simulink model "TBRe18_ECU_V6"  (R2015b)
settings: Solver=FixedStepDiscrete  SolverMode=SingleTasking  StartTime=0.0  StopTime=inf  FixedStep=0.0001  RelTol=1e-3
PostLoadFcn:
  | model_init();
libraries: simulink x20, simulink_extras x1
(part 1 of 4)
settings Model: Creator=agf25  LastModifiedBy=William
settings OptimizationCC: DefaultParameterBehavior=Inlined  EfficientFloat2IntCast=on
settings RTWCC: SystemTargetFile=nsi_mpc.tlc  MakeCommand=nsi_make  TemplateMakefile=nsi_mpc.tmf  Description=RTW Coder for MUXLAB4
settings STFCustomTargetCC: ConcurrentExecutionCompliant=off  GeneratePreprocessorConditionals=Use local settings  MATLABClassNameForMDSCustomization=Simulink.SoftwareTarget.TargetSpecificTriggerConfigurationBase  CPPClassGenCompliant=off  SystemTargetFile=nsi_mpc.tlc

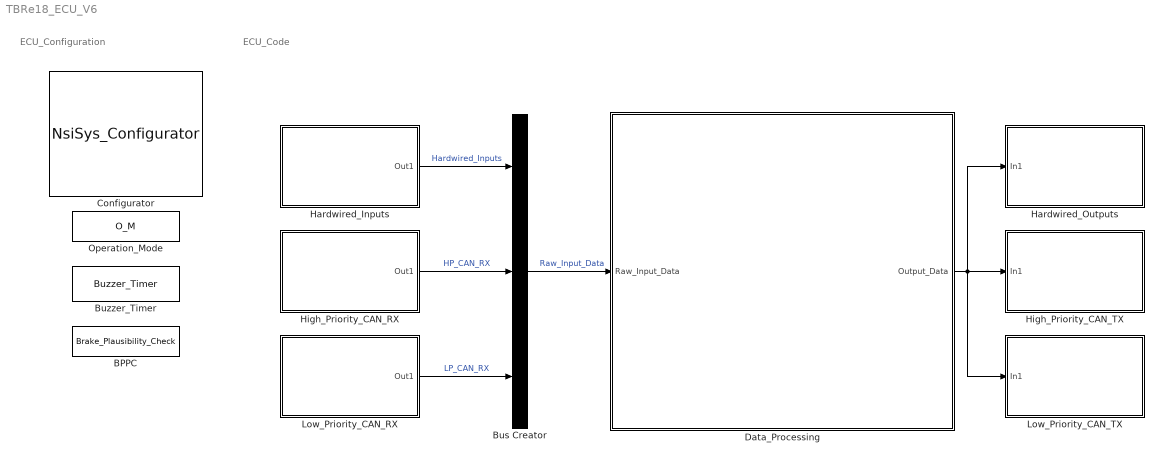
== system TBRe18_ECU_V6 ==
  note: ECU_Code
  note: ECU_Configuration
  BPPC : DataStoreMemory  DataStoreName=Brake_Plausibility_Check  ReadBeforeWriteMsg=warning  WriteAfterWriteMsg=warning  WriteAfterReadMsg=warning  OutDataTypeStr=boolean
  Bus Creator : BusCreator  Inputs=3
  Buzzer_Timer : DataStoreMemory  DataStoreName=Buzzer_Timer  ReadBeforeWriteMsg=warning  WriteAfterWriteMsg=warning  WriteAfterReadMsg=warning
  Configurator : S-Function  FunctionName=NsiSys_Configurator  Parameters=main,io,nbof_can,can,ccp,flash,nbof_lin,lin,tasks  SFunctionDeploymentMode=off  EnableBusSupport=off  mask(Configurator block){main=Config description;01/01/2011;0, io=2.5;0;1;1;0;0;1;1;1, nbof_can=5, can=1;HIGH_SPEED;500Kbps;120 Ohm;C:\Users\William\Documents\ECU\DBC\TBRe18_DBC_V1.dbc;0;1;1;HIGH_SPEED;500Kbps;120 Ohm;C:\Users\William\Documents\ECU\DBC\TBRe18_DBC_V1.dbc;0;1;0;HIGH_SPEED;500Kbps;120 Ohm;C:\Users\l\Desktop\FYP\ECU\DBC\TBRe_DBC_V2.dbc;0;0;0;HIGH_SPEED;500Kbps;120 Ohm;D:\TOOLS\MUXLINK\R2011b\MUXlink\misc\j1939_adapt.dbc;0;1;0;HIGH_SPEED;1000Kbps;No;D:\TOOLS\MUXLINK\R2011b\MUXlink\misc\BASE_CAN_MUXLAB4.dbc;0;0, ccp=0;0x100;0x200;0;0;0x0;0x0;0;0x13, flash=Vehicle_STATE;No;Unsigned Byte;0;1;Operational_STATE;No;Unsigned Byte;0;1;Buzzer_time;No;Unsigned Byte;254;1;Buzzer_on;No;Boolean;1;1;reset_MEM;No;Boolean;0;1;TC_Slip_target;No;Unsigned Byte;5;1;TC_P_Gain;No;Unsigned Byte;1;1;TC_I_Gain;No;Unsigned Byte;1;1;TC_Offset;No;Signed Byte;0;1;DM_Mode;No;Unsigned Byte;0;1;DM_I_Gain;No;Unsigned Byte;1;1;IMD_MEM;No;Boolean;0;1;status_vehcle_LV;No;Boolean;0;1;status_vehcle_HV;No;Boolean;0;1;status_BMS;No;Boolean;0;1;status_IMD;No;Boolean;0;1;status_APPC;No;Boolean;0;1;status_APPS_BPPC;No;Boolean;0;1;status_RTD;No;Boolean;0;1;status_TC;No;Boolean;0;1;status_power_lim;No;Boolean;0;1;status_torque_derate;No;Boolean;0;1;status_tyre_radius;No;Unsigned Byte;22;1;power_limit;No;Unsigned Byte;30;1;torque_limit;No;Unsigned Byte;80;1, nbof_lin=2, lin=0;D:\TOOLS\MUXLINK\R2011b\MUXlink\misc\lindb.ldf;1;0.0;0.0;0.000;0.000;0.000000;0,0;0;D:\TOOLS\MUXLINK\R2011b\MUXlink\misc\lindb.ldf;1;0.0;0.0;0.000;0.000;0.000000;0,0, tasks=Data_Processing;[0.100];Hardwired_Inputs;[0.1];Hardwired_Outputs;[0.1];High_Priority_CAN_RX;[0.1];High_Priority_CAN_TX;[0.1];Low_Priority_CAN_RX;[0.1];Low_Priority_CAN_TX;[0.1]}
      mask prompts: nbof_can "nbof can"
      mask help: This block permits to set general parameters to use a MUXlink model
      mask init:
      | NsiSys_Configurator_InitializationFcn();
      settings: OpenFcn=NsiSys_Configurator_OpenFcn();
      mask Help:
      | eval('block=get_param(gcb, ''RTWdata'');')
      | web([docroot '\toolbox\MUXlink\html\blocks/' block.MUXlink_BlockType '.html'])
      mask Callback main: NsiSys_Configurator_ApplyFcn(1);
      mask Callback io: NsiSys_Configurator_ApplyFcn(2);
      mask Callback nbof_can: NsiSys_Configurator_ApplyFcn(3);
      mask Callback can: NsiSys_Configurator_ApplyFcn(4);
      mask Callback ccp: NsiSys_Configurator_ApplyFcn(5);
      mask Callback flash: NsiSys_Configurator_ApplyFcn(6);
      mask Callback nbof_lin: NsiSys_Configurator_ApplyFcn(7);
      mask Callback lin: NsiSys_Configurator_ApplyFcn(8);
      mask Callback tasks: NsiSys_Configurator_ApplyFcn(9);
      mask Display: image(imread('MUXLAB4.bmp'));text(0.5, 0.2, '', 'horizontalAlignment', 'center', 'verticalAlignment', 'base');
  Data_Processing : Subsystem  TreatAsAtomicUnit=on  SystemSampleTime=[0.100]  RTWFcnName=Data_Processing  RTWFileName=FileTaskFcn
      mask init:
      | NsiSys_SubSystemTask_InitializationFcn();
      settings: OpenFcn=NsiSys_SubSystemTask_OpenFcn();  RTWSystemCode=Nonreusable function  RTWFcnNameOpts=User specified  RTWFileNameOpts=Use function name
      mask Display: image(imread('nsi.bmp'));text(0.45, 0.9, 'task()');plot([0.05 0.05 0.05 0.05 0.05 0.05 0.05 0.05 0.05 0.05]);fprintf('Data_Processing\n/ 100.0ms / 30.0ms /\nEvent');
  Hardwired_Inputs : Subsystem  TreatAsAtomicUnit=on  SystemSampleTime=[0.1]  RTWFcnName=Hardwired_Inputs  RTWFileName=FileTaskFcn
      mask init:
      | NsiSys_SubSystemTask_InitializationFcn();
      settings: OpenFcn=NsiSys_SubSystemTask_OpenFcn();  RTWSystemCode=Nonreusable function  RTWFcnNameOpts=User specified  RTWFileNameOpts=Use function name
      mask Display: image(imread('nsi.bmp'));text(0.45, 0.9, 'task()');plot([0.05 0.05 0.05 0.05 0.05 0.05 0.05 0.05 0.05 0.05]);fprintf('Hardwired_Inputs\n/ 100.0ms / 40.0ms /\nEvent');
  Hardwired_Outputs : Subsystem  TreatAsAtomicUnit=on  SystemSampleTime=[0.1]  RTWFcnName=Hardwired_Outputs  RTWFileName=FileTaskFcn
      mask init:
      | NsiSys_SubSystemTask_InitializationFcn();
      settings: OpenFcn=NsiSys_SubSystemTask_OpenFcn();  RTWSystemCode=Nonreusable function  RTWFcnNameOpts=User specified  RTWFileNameOpts=Use function name
      mask Display: image(imread('nsi.bmp'));text(0.45, 0.9, 'task()');plot([0.05 0.05 0.05 0.05 0.05 0.05 0.05 0.05 0.05 0.05]);fprintf('Hardwired_Outputs\n/ 100.0ms / 30.0ms /\nEvent');
  High_Priority_CAN_RX : Subsystem  TreatAsAtomicUnit=on  SystemSampleTime=[0.1]  RTWFcnName=High_Priority_CAN_RX  RTWFileName=FileTaskFcn
      mask init:
      | NsiSys_SubSystemTask_InitializationFcn();
      settings: OpenFcn=NsiSys_SubSystemTask_OpenFcn();  RTWSystemCode=Nonreusable function  RTWFcnNameOpts=User specified  RTWFileNameOpts=Use function name
      mask Display: image(imread('nsi.bmp'));text(0.45, 0.9, 'task()');plot([0.05 0.05 0.05 0.05 0.05 0.05 0.05 0.05 0.05 0.05]);fprintf('High_Priority_CAN_RX\n/ 100.0ms / 30.0ms /\nEvent');
  High_Priority_CAN_TX : Subsystem  TreatAsAtomicUnit=on  SystemSampleTime=[0.1]  RTWFcnName=High_Priority_CAN_TX  RTWFileName=FileTaskFcn
      mask init:
      | NsiSys_SubSystemTask_InitializationFcn();
      settings: OpenFcn=NsiSys_SubSystemTask_OpenFcn();  RTWSystemCode=Nonreusable function  RTWFcnNameOpts=User specified  RTWFileNameOpts=Use function name
      mask Display: image(imread('nsi.bmp'));text(0.45, 0.9, 'task()');plot([0.05 0.05 0.05 0.05 0.05 0.05 0.05 0.05 0.05 0.05]);fprintf('High_Priority_CAN_TX\n/ 100.0ms / 30.0ms /\nEvent');
  Low_Priority_CAN_RX : Subsystem  TreatAsAtomicUnit=on  SystemSampleTime=[0.1]  RTWFcnName=Low_Priority_CAN_RX  RTWFileName=FileTaskFcn
      mask init:
      | NsiSys_SubSystemTask_InitializationFcn();
      settings: OpenFcn=NsiSys_SubSystemTask_OpenFcn();  RTWSystemCode=Nonreusable function  RTWFcnNameOpts=User specified  RTWFileNameOpts=Use function name
      mask Display: image(imread('nsi.bmp'));text(0.45, 0.9, 'task()');plot([0.05 0.05 0.05 0.05 0.05 0.05 0.05 0.05 0.05 0.05]);fprintf('Low_Priority_CAN_RX\n/ 100.0ms / 50.0ms /\nEvent');
  Low_Priority_CAN_TX : Subsystem  TreatAsAtomicUnit=on  SystemSampleTime=[0.1]  RTWFcnName=Low_Priority_CAN_TX  RTWFileName=FileTaskFcn
      mask init:
      | NsiSys_SubSystemTask_InitializationFcn();
      settings: OpenFcn=NsiSys_SubSystemTask_OpenFcn();  RTWSystemCode=Nonreusable function  RTWFcnNameOpts=User specified  RTWFileNameOpts=Use function name
      mask Display: image(imread('nsi.bmp'));text(0.45, 0.9, 'task()');plot([0.05 0.05 0.05 0.05 0.05 0.05 0.05 0.05 0.05 0.05]);fprintf('Low_Priority_CAN_TX\n/ 100.0ms / 30.0ms /\nEvent');
  Operation_Mode : DataStoreMemory  DataStoreName=O_M  ReadBeforeWriteMsg=warning  WriteAfterWriteMsg=warning  WriteAfterReadMsg=warning
  wires:
  Low_Priority_CAN_RX/1(Out1) -> Bus Creator/3  "LP_CAN_RX"
  High_Priority_CAN_RX/1(Out1) -> Bus Creator/2  "HP_CAN_RX"
  Hardwired_Inputs/1(Out1) -> Bus Creator/1  "Hardwired_Inputs"
  Bus Creator/1 -> Data_Processing/1(Raw_Input_Data)  "Raw_Input_Data"
  Data_Processing/1(Output_Data) -> Low_Priority_CAN_TX/1(In1), High_Priority_CAN_TX/1(In1), Hardwired_Outputs/1(In1)

== system TBRe18_ECU_V6/Data_Processing ==
  note: Data_Processing
  Raw_Input_Data : Inport
  Diagnostics : Subsystem
  Init : Subsystem  mask(System Initialize){}
      mask help: Add code to a systems Initialize function
      settings: CopyFcn=cccopyfcn(gcb)  OpenFcn=ccopenfcn('System Initialize Function')
      mask Help: This block contains text fields to insert custom user code sections at the declaration, execution and exit sections of the systems initialize function.  By placing this block inside a subsytem, the custom user code will appear in that subsystems function.
      mask Display: disp('I()')
  Signal Conversion : SignalConversion
  Task : S-Function  FunctionName=NsiSys_TaskREF  Parameters=task_initialised,task_periodic, task_sampletime,task_name,task_event,task_offset  SFunctionDeploymentMode=off  EnableBusSupport=off  mask(task definition){task_initialised=on, task_periodic=on, task_sampletime=[0.100], task_offset=0.03, task_name=Data_Processing, task_event=on}
      mask prompts: task_initialised "task initialised"; task_periodic "Is Periodic"; task_sampletime "Task sample time"; task_offset "Task Offset"; task_name "Task name"; task_event "Is event"
      mask help:
      | Permit to provide all parameters associated to a MUXLINK task.
      | Task can be executed periodicaly and/or on event detection.
      | If task is periodic:
      | Task sample time specify the execution period in mS [0.001   6000]
      | Task Offset specify the offset applied to the execution period
      | Task Offset < Task sample time
      mask init:
      | NsiSys_TaskREF_InitializationFcn();
      settings: OpenFcn=NsiSys_Task_OpenFcn();
      mask Callback task_initialised: NsiSys_TaskREF_ApplyFcn(1);
      mask Callback task_periodic: NsiSys_TaskREF_ApplyFcn(2);
      mask Callback task_sampletime: NsiSys_TaskREF_ApplyFcn(3);
      mask Callback task_offset: NsiSys_TaskREF_ApplyFcn(6);
      mask Callback task_name: NsiSys_TaskREF_ApplyFcn(4);
      mask Callback task_event: NsiSys_TaskREF_ApplyFcn(5);
      mask Display: text(0.5, 0.8, 't()', 'horizontalAlignment', 'center', 'verticalAlignment', 'base');text(0.5, 0.2, '/ 100.0ms / 30.0ms /', 'horizontalAlignment', 'center', 'verticalAlignment', 'base');text(0.5, 0.4, 'Event', 'horizontalAlignment', 'center', 'verticalAlignment', 'base');
  Vehicle_Functionality : Subsystem
  Output_Data : Outport
  wires:
  Raw_Input_Data/1 -> Signal Conversion/1
  Diagnostics/1(Input_Data_Bus) -> Vehicle_Functionality/1(Input_Data)
  Signal Conversion/1 -> Diagnostics/1(Raw_Input_Data)
  Vehicle_Functionality/1(Output_Data_Bus) -> Output_Data/1

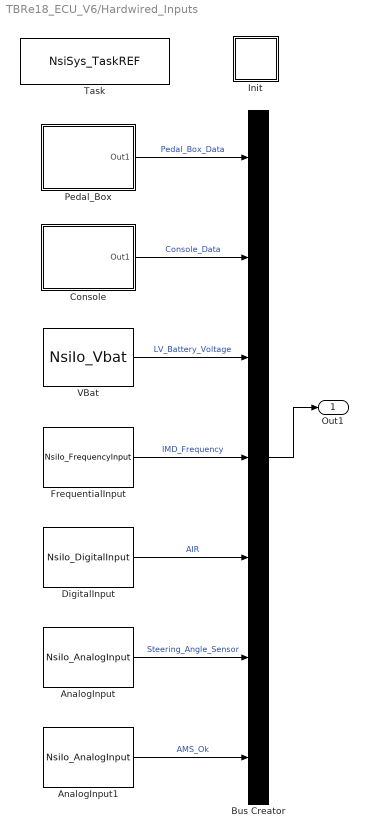
== system TBRe18_ECU_V6/Hardwired_Inputs ==
  AnalogInput : S-Function  FunctionName=NsiIo_AnalogInput  Parameters=channel  SFunctionDeploymentMode=off  EnableBusSupport=off  mask(MUXlink I/O Analog Input){channel=4}
      mask prompts: channel "Channel ?"
      mask help: Read analogic input from ADC channel.
      mask init:
      | NsiIo_AnalogInput_InitializationFcn();
      settings: OpenFcn=NsiIo_AnalogInput_OpenFcn();
      mask Help:
      | eval('block=get_param(gcb, ''RTWdata'');')
      | web([docroot '\toolbox\MUXlink\html\blocks/' block.MUXlink_BlockType '.html'])
      mask Callback channel: NsiIo_AnalogInput_ApplyFcn(1);
      mask Display: image(imread('nsi.bmp'));text(0.5, 0.2, 'AnalogInput_4', 'horizontalAlignment', 'center', 'verticalAlignment', 'base');plot([0.05 0.05 0.05 0.05 0.05 0.05 0.05 0.05 0.05 0.05]);port_label('output', 1, 'B4');
  AnalogInput1 : S-Function  FunctionName=NsiIo_AnalogInput  Parameters=channel  SFunctionDeploymentMode=off  EnableBusSupport=off  mask(MUXlink I/O Analog Input){channel=7}
      mask prompts: channel "Channel ?"
      mask help: Read analogic input from ADC channel.
      mask init:
      | NsiIo_AnalogInput_InitializationFcn();
      settings: OpenFcn=NsiIo_AnalogInput_OpenFcn();
      mask Help:
      | eval('block=get_param(gcb, ''RTWdata'');')
      | web([docroot '\toolbox\MUXlink\html\blocks/' block.MUXlink_BlockType '.html'])
      mask Callback channel: NsiIo_AnalogInput_ApplyFcn(1);
      mask Display: image(imread('nsi.bmp'));text(0.5, 0.2, 'AnalogInput_7', 'horizontalAlignment', 'center', 'verticalAlignment', 'base');plot([0.05 0.05 0.05 0.05 0.05 0.05 0.05 0.05 0.05 0.05]);port_label('output', 1, 'D3');
  Bus Creator : BusCreator  Inputs=7
  Console : Subsystem
  DigitalInput : S-Function  FunctionName=NsiIo_DigitalInput  Parameters=channel,is_trigger,typeof_trigger,is_wakeup,wakeup_level  SFunctionDeploymentMode=off  EnableBusSupport=off  mask(MUXlink I/O Digital Input){channel=1, is_trigger=off, typeof_trigger=Either, is_wakeup=off, wakeup_level=Low level}
      mask prompts: channel "Channel ?"; is_trigger "Trigger ?"; typeof_trigger "Type of Trigger ?"; is_wakeup "Wake-up ?"; wakeup_level "Wake-up level ?"
      mask help: Read digital input from I/O channel.
      mask init:
      | NsiIo_DigitalInput_InitializationFcn();
      settings: OpenFcn=NsiIo_DigitalInput_OpenFcn();
      mask Help:
      | eval('block=get_param(gcb, ''RTWdata'');')
      | web([docroot '\toolbox\MUXlink\html\blocks/' block.MUXlink_BlockType '.html'])
      mask Callback channel: NsiIo_DigitalInput_ApplyFcn(1);
      mask Callback is_trigger: NsiIo_DigitalInput_ApplyFcn(2);
      mask TypeOptions typeof_trigger: Rising | Falling | Either
      mask Callback typeof_trigger: NsiIo_DigitalInput_ApplyFcn(3);
      mask Callback is_wakeup: NsiIo_DigitalInput_ApplyFcn(4);
      mask TypeOptions wakeup_level: Low level | High level
      mask Callback wakeup_level: NsiIo_DigitalInput_ApplyFcn(5);
      mask Display: image(imread('nsi.bmp'));text(0.5, 0.2, 'DigitalInput_1', 'horizontalAlignment', 'center', 'verticalAlignment', 'base');plot([0.05 0.05 0.05 0.05 0.05 0.05 0.05 0.05 0.05 0.05]);port_label('output', 1, 'Ground : A1');
  FrequentialInput : S-Function  FunctionName=NsiIo_FrequencyInput  Parameters=channel,max_freq,is_digital_input  SFunctionDeploymentMode=off  EnableBusSupport=off  mask(MUXlink I/O Frequential Input){channel=3, max_freq=10KHZ, is_digital_input=off}
      mask prompts: channel "Channel ?"; max_freq "Max Frequency ?"; is_digital_input "Used as Digital Input ?"
      mask help: Read Frequency from I/O Frequential Input.
      mask init:
      | NsiIo_FrequencyInput_InitializationFcn();
      settings: OpenFcn=NsiIo_FrequencyInput_OpenFcn();
      mask Help:
      | eval('block=get_param(gcb, ''RTWdata'');')
      | web([docroot '\toolbox\MUXlink\html\blocks/' block.MUXlink_BlockType '.html'])
      mask Callback channel: NsiIo_FrequencyInput_ApplyFcn(1);
      mask TypeOptions max_freq: 10KHZ | 100KHZ
      mask Callback max_freq: NsiIo_FrequencyInput_ApplyFcn(2);
      mask Callback is_digital_input: NsiIo_FrequencyInput_ApplyFcn(3);
      mask Display: image(imread('nsi.bmp'));text(0.5, 0.2, 'FrequencyInput_3  10KHZ', 'horizontalAlignment', 'center', 'verticalAlignment', 'base');plot([0.05 0.05 0.05 0.05 0.05 0.05 0.05 0.05 0.05 0.05]);port_label('output', 1, 'Freq C3');
  Init : Subsystem  mask(System Initialize){}
      mask help: Add code to a systems Initialize function
      settings: CopyFcn=cccopyfcn(gcb)  OpenFcn=ccopenfcn('System Initialize Function')
      mask Help: This block contains text fields to insert custom user code sections at the declaration, execution and exit sections of the systems initialize function.  By placing this block inside a subsytem, the custom user code will appear in that subsystems function.
      mask Display: disp('I()')
  Pedal_Box : Subsystem
  Task : S-Function  FunctionName=NsiSys_TaskREF  Parameters=task_initialised,task_periodic, task_sampletime,task_name,task_event,task_offset  SFunctionDeploymentMode=off  EnableBusSupport=off  mask(task definition){task_initialised=on, task_periodic=on, task_sampletime=[0.1], task_offset=0.04, task_name=Hardwired_Inputs, task_event=on}
      mask prompts: task_initialised "task initialised"; task_periodic "Is Periodic"; task_sampletime "Task sample time"; task_offset "Task Offset"; task_name "Task name"; task_event "Is event"
      mask help:
      | Permit to provide all parameters associated to a MUXLINK task.
      | Task can be executed periodicaly and/or on event detection.
      | If task is periodic:
      | Task sample time specify the execution period in mS [0.001   6000]
      | Task Offset specify the offset applied to the execution period
      | Task Offset < Task sample time
      mask init:
      | NsiSys_TaskREF_InitializationFcn();
      settings: OpenFcn=NsiSys_Task_OpenFcn();
      mask Callback task_initialised: NsiSys_TaskREF_ApplyFcn(1);
      mask Callback task_periodic: NsiSys_TaskREF_ApplyFcn(2);
      mask Callback task_sampletime: NsiSys_TaskREF_ApplyFcn(3);
      mask Callback task_offset: NsiSys_TaskREF_ApplyFcn(6);
      mask Callback task_name: NsiSys_TaskREF_ApplyFcn(4);
      mask Callback task_event: NsiSys_TaskREF_ApplyFcn(5);
      mask Display: text(0.5, 0.8, 't()', 'horizontalAlignment', 'center', 'verticalAlignment', 'base');text(0.5, 0.2, '/ 100.0ms / 40.0ms /', 'horizontalAlignment', 'center', 'verticalAlignment', 'base');text(0.5, 0.4, 'Event', 'horizontalAlignment', 'center', 'verticalAlignment', 'base');
  VBat : S-Function  FunctionName=NsiIo_Vbat  SFunctionDeploymentMode=off  EnableBusSupport=off  mask(MUXlink I/O VBat){}
      mask help: Battery Voltage
      mask init:
      | NsiIo_Vbat_InitializationFcn();
      settings: OpenFcn=NsiIo_Vbat_OpenFcn();
      mask Help:
      | eval('block=get_param(gcb, ''RTWdata'');')
      | web([docroot '\toolbox\MUXlink\html\blocks/' block.MUXlink_BlockType '.html'])
      mask Display: image(imread('nsi.bmp'));text(0.5, 0.2, 'I/O VBat', 'horizontalAlignment', 'center', 'verticalAlignment', 'base');plot([0.05 0.05 0.05 0.05 0.05 0.05 0.05 0.05 0.05 0.05]);port_label('output', 1, 'Voltage');
  Out1 : Outport
  wires:
  Pedal_Box/1(Out1) -> Bus Creator/1  "Pedal_Box_Data"
  Console/1(Out1) -> Bus Creator/2  "Console_Data"
  Bus Creator/1 -> Out1/1
  VBat/1 -> Bus Creator/3  "LV_Battery_Voltage"
  FrequentialInput/1 -> Bus Creator/4  "IMD_Frequency"
  DigitalInput/1 -> Bus Creator/5  "AIR"
  AnalogInput/1 -> Bus Creator/6  "Steering_Angle_Sensor"
  AnalogInput1/1 -> Bus Creator/7  "AMS_Ok"

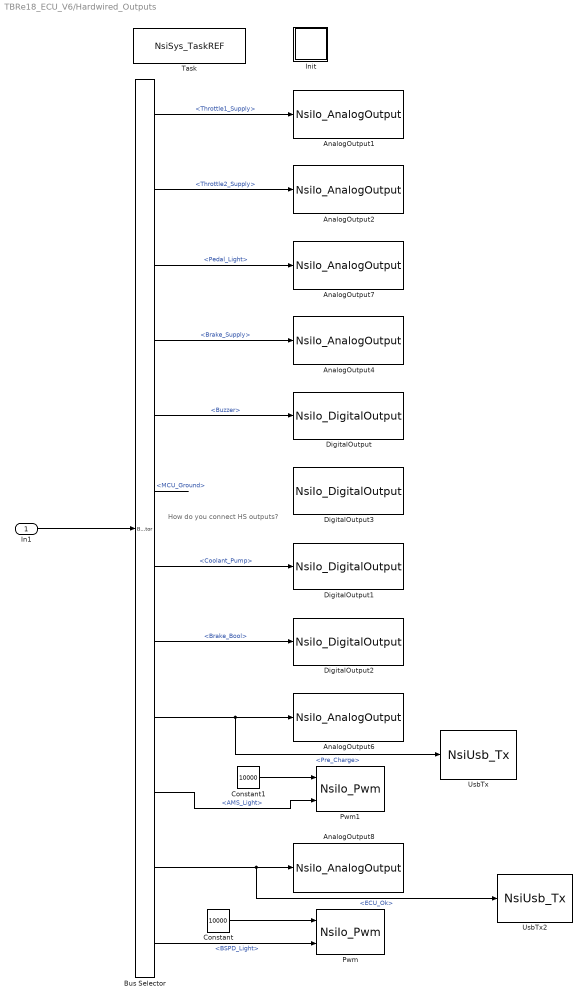
== system TBRe18_ECU_V6/Hardwired_Outputs ==
  note: How do you connect HS outputs?
  In1 : Inport
  AnalogOutput1 : S-Function  FunctionName=NsiIo_AnalogOutput  Parameters=Channel,Feedback  SFunctionDeploymentMode=off  EnableBusSupport=off  mask(MUXlink I/O Analog Output){Channel=3, Feedback=off}
      mask prompts: Channel "Channel ?"; Feedback "Read Back Analog out"
      mask help: Write Analog Output onto DAC channel.
      mask init:
      | NsiIo_AnalogOutput_InitializationFcn();
      settings: OpenFcn=NsiIo_AnalogOutput_OpenFcn();
      mask Help:
      | eval('block=get_param(gcb, ''RTWdata'');')
      | web([docroot '\toolbox\MUXlink\html\blocks/' block.MUXlink_BlockType '.html'])
      mask Callback Channel: NsiIo_AnalogOutput_ApplyFcn(1);
      mask Display: image(imread('nsi.bmp'));text(0.5, 0.2, 'AnalogOutput_3', 'horizontalAlignment', 'center', 'verticalAlignment', 'base');plot([0.05 0.05 0.05 0.05 0.05 0.05 0.05 0.05 0.05 0.05]);port_label('input', 1, 'F1');
  AnalogOutput2 : S-Function  FunctionName=NsiIo_AnalogOutput  Parameters=Channel,Feedback  SFunctionDeploymentMode=off  EnableBusSupport=off  mask(MUXlink I/O Analog Output){Channel=4, Feedback=off}
      mask prompts: Channel "Channel ?"; Feedback "Read Back Analog out"
      mask help: Write Analog Output onto DAC channel.
      mask init:
      | NsiIo_AnalogOutput_InitializationFcn();
      settings: OpenFcn=NsiIo_AnalogOutput_OpenFcn();
      mask Help:
      | eval('block=get_param(gcb, ''RTWdata'');')
      | web([docroot '\toolbox\MUXlink\html\blocks/' block.MUXlink_BlockType '.html'])
      mask Callback Channel: NsiIo_AnalogOutput_ApplyFcn(1);
      mask Display: image(imread('nsi.bmp'));text(0.5, 0.2, 'AnalogOutput_4', 'horizontalAlignment', 'center', 'verticalAlignment', 'base');plot([0.05 0.05 0.05 0.05 0.05 0.05 0.05 0.05 0.05 0.05]);port_label('input', 1, 'F2');
  AnalogOutput4 : S-Function  FunctionName=NsiIo_AnalogOutput  Parameters=Channel,Feedback  SFunctionDeploymentMode=off  EnableBusSupport=off  mask(MUXlink I/O Analog Output){Channel=5, Feedback=off}
      mask prompts: Channel "Channel ?"; Feedback "Read Back Analog out"
      mask help: Write Analog Output onto DAC channel.
      mask init:
      | NsiIo_AnalogOutput_InitializationFcn();
      settings: OpenFcn=NsiIo_AnalogOutput_OpenFcn();
      mask Help:
      | eval('block=get_param(gcb, ''RTWdata'');')
      | web([docroot '\toolbox\MUXlink\html\blocks/' block.MUXlink_BlockType '.html'])
      mask Callback Channel: NsiIo_AnalogOutput_ApplyFcn(1);
      mask Display: image(imread('nsi.bmp'));text(0.5, 0.2, 'AnalogOutput_5', 'horizontalAlignment', 'center', 'verticalAlignment', 'base');plot([0.05 0.05 0.05 0.05 0.05 0.05 0.05 0.05 0.05 0.05]);port_label('input', 1, 'F3');
  AnalogOutput6 : S-Function  FunctionName=NsiIo_AnalogOutput  Parameters=Channel,Feedback  SFunctionDeploymentMode=off  EnableBusSupport=off  mask(MUXlink I/O Analog Output){Channel=7, Feedback=off}
      mask prompts: Channel "Channel ?"; Feedback "Read Back Analog out"
      mask help: Write Analog Output onto DAC channel.
      mask init:
      | NsiIo_AnalogOutput_InitializationFcn();
      settings: OpenFcn=NsiIo_AnalogOutput_OpenFcn();
      mask Help:
      | eval('block=get_param(gcb, ''RTWdata'');')
      | web([docroot '\toolbox\MUXlink\html\blocks/' block.MUXlink_BlockType '.html'])
      mask Callback Channel: NsiIo_AnalogOutput_ApplyFcn(1);
      mask Display: image(imread('nsi.bmp'));text(0.5, 0.2, 'AnalogOutput_7', 'horizontalAlignment', 'center', 'verticalAlignment', 'base');plot([0.05 0.05 0.05 0.05 0.05 0.05 0.05 0.05 0.05 0.05]);port_label('input', 1, 'A2');
  AnalogOutput7 : S-Function  FunctionName=NsiIo_AnalogOutput  Parameters=Channel,Feedback  SFunctionDeploymentMode=off  EnableBusSupport=off  mask(MUXlink I/O Analog Output){Channel=6, Feedback=off}
      mask prompts: Channel "Channel ?"; Feedback "Read Back Analog out"
      mask help: Write Analog Output onto DAC channel.
      mask init:
      | NsiIo_AnalogOutput_InitializationFcn();
      settings: OpenFcn=NsiIo_AnalogOutput_OpenFcn();
      mask Help:
      | eval('block=get_param(gcb, ''RTWdata'');')
      | web([docroot '\toolbox\MUXlink\html\blocks/' block.MUXlink_BlockType '.html'])
      mask Callback Channel: NsiIo_AnalogOutput_ApplyFcn(1);
      mask Display: image(imread('nsi.bmp'));text(0.5, 0.2, 'AnalogOutput_6', 'horizontalAlignment', 'center', 'verticalAlignment', 'base');plot([0.05 0.05 0.05 0.05 0.05 0.05 0.05 0.05 0.05 0.05]);port_label('input', 1, 'F4');
  AnalogOutput8 : S-Function  FunctionName=NsiIo_AnalogOutput  Parameters=Channel,Feedback  SFunctionDeploymentMode=off  EnableBusSupport=off  mask(MUXlink I/O Analog Output){Channel=2, Feedback=off}
      mask prompts: Channel "Channel ?"; Feedback "Read Back Analog out"
      mask help: Write Analog Output onto DAC channel.
      mask init:
      | NsiIo_AnalogOutput_InitializationFcn();
      settings: OpenFcn=NsiIo_AnalogOutput_OpenFcn();
      mask Help:
      | eval('block=get_param(gcb, ''RTWdata'');')
      | web([docroot '\toolbox\MUXlink\html\blocks/' block.MUXlink_BlockType '.html'])
      mask Callback Channel: NsiIo_AnalogOutput_ApplyFcn(1);
      mask Display: image(imread('nsi.bmp'));text(0.5, 0.2, 'AnalogOutput_2', 'horizontalAlignment', 'center', 'verticalAlignment', 'base');plot([0.05 0.05 0.05 0.05 0.05 0.05 0.05 0.05 0.05 0.05]);port_label('input', 1, 'E4');
  Bus Selector : BusSelector  OutputSignals=Hardwired_Output_Data.Throttle1_Supply,Hardwired_Output_Data.Throttle2_Supply,Hardwired_Output_Data.Pedal_Light,Hardwired_Output_Data.Brake_Supply,Vehicle_Operation_Data.Buzzer,Hardwired_Output_Data.MCU_Ground,Hardwired_Output_Data.Coolant_Pump,Hardwired_Output_Data.Brake_Bool,Hardwired_Output_Data.Pre_Charge,Hardwired_Output_Data.AMS_Light,Hardwired_Output_Data.ECU_Ok,Hardwired_Output_Data.BSPD_Light
  Constant : Constant  Value=10000  OutDataTypeStr=uint32
  Constant1 : Constant  Value=10000  OutDataTypeStr=uint32
  DigitalOutput : S-Function  FunctionName=NsiIo_DigitalOutput  Parameters=channel,side,feedback  SFunctionDeploymentMode=off  EnableBusSupport=off  mask(MUXlink I/O Digital Output){channel=3, side=High, feedback=off}
      mask prompts: channel "Channel ?"; side "Side ?"; feedback "With feedback ?"
      mask help: Write Digital Output onto I/O channel.
      mask init:
      | NsiIo_DigitalOutput_InitializationFcn();
      settings: OpenFcn=NsiIo_DigitalOutput_OpenFcn();
      mask Help:
      | eval('block=get_param(gcb, ''RTWdata'');')
      | web([docroot '\toolbox\MUXlink\html\blocks/' block.MUXlink_BlockType '.html'])
      mask Callback channel: NsiIo_DigitalOutput_ApplyFcn(1);
      mask TypeOptions side: High | Low
      mask Callback side: NsiIo_DigitalOutput_ApplyFcn(2);
      mask Callback feedback: NsiIo_DigitalOutput_ApplyFcn(3);
      mask Display: image(imread('nsi.bmp'));text(0.5, 0.2, 'DigitalOutput_3', 'horizontalAlignment', 'center', 'verticalAlignment', 'base');plot([0.05 0.05 0.05 0.05 0.05 0.05 0.05 0.05 0.05 0.05]);port_label('input', 1, 'L3 : High Side');
  DigitalOutput1 : S-Function  FunctionName=NsiIo_DigitalOutput  Parameters=channel,side,feedback  SFunctionDeploymentMode=off  EnableBusSupport=off  mask(MUXlink I/O Digital Output){channel=1, side=High, feedback=off}
      mask prompts: channel "Channel ?"; side "Side ?"; feedback "With feedback ?"
      mask help: Write Digital Output onto I/O channel.
      mask init:
      | NsiIo_DigitalOutput_InitializationFcn();
      settings: OpenFcn=NsiIo_DigitalOutput_OpenFcn();
      mask Help:
      | eval('block=get_param(gcb, ''RTWdata'');')
      | web([docroot '\toolbox\MUXlink\html\blocks/' block.MUXlink_BlockType '.html'])
      mask Callback channel: NsiIo_DigitalOutput_ApplyFcn(1);
      mask TypeOptions side: High | Low
      mask Callback side: NsiIo_DigitalOutput_ApplyFcn(2);
      mask Callback feedback: NsiIo_DigitalOutput_ApplyFcn(3);
      mask Display: image(imread('nsi.bmp'));text(0.5, 0.2, 'DigitalOutput_1', 'horizontalAlignment', 'center', 'verticalAlignment', 'base');plot([0.05 0.05 0.05 0.05 0.05 0.05 0.05 0.05 0.05 0.05]);port_label('input', 1, 'G2 : High Side');
  DigitalOutput2 : S-Function  FunctionName=NsiIo_DigitalOutput  Parameters=channel,side,feedback  SFunctionDeploymentMode=off  EnableBusSupport=off  mask(MUXlink I/O Digital Output){channel=2, side=High, feedback=off}
      mask prompts: channel "Channel ?"; side "Side ?"; feedback "With feedback ?"
      mask help: Write Digital Output onto I/O channel.
      mask init:
      | NsiIo_DigitalOutput_InitializationFcn();
      settings: OpenFcn=NsiIo_DigitalOutput_OpenFcn();
      mask Help:
      | eval('block=get_param(gcb, ''RTWdata'');')
      | web([docroot '\toolbox\MUXlink\html\blocks/' block.MUXlink_BlockType '.html'])
      mask Callback channel: NsiIo_DigitalOutput_ApplyFcn(1);
      mask TypeOptions side: High | Low
      mask Callback side: NsiIo_DigitalOutput_ApplyFcn(2);
      mask Callback feedback: NsiIo_DigitalOutput_ApplyFcn(3);
      mask Display: image(imread('nsi.bmp'));text(0.5, 0.2, 'DigitalOutput_2', 'horizontalAlignment', 'center', 'verticalAlignment', 'base');plot([0.05 0.05 0.05 0.05 0.05 0.05 0.05 0.05 0.05 0.05]);port_label('input', 1, 'G3 : High Side');
  DigitalOutput3 : S-Function  FunctionName=NsiIo_DigitalOutput  Parameters=channel,side,feedback  SFunctionDeploymentMode=off  EnableBusSupport=off  mask(MUXlink I/O Digital Output){channel=1, side=Low, feedback=off}
      mask prompts: channel "Channel ?"; side "Side ?"; feedback "With feedback ?"
      mask help: Write Digital Output onto I/O channel.
      mask init:
      | NsiIo_DigitalOutput_InitializationFcn();
      settings: OpenFcn=NsiIo_DigitalOutput_OpenFcn();
      mask Help:
      | eval('block=get_param(gcb, ''RTWdata'');')
      | web([docroot '\toolbox\MUXlink\html\blocks/' block.MUXlink_BlockType '.html'])
      mask Callback channel: NsiIo_DigitalOutput_ApplyFcn(1);
      mask TypeOptions side: High | Low
      mask Callback side: NsiIo_DigitalOutput_ApplyFcn(2);
      mask Callback feedback: NsiIo_DigitalOutput_ApplyFcn(3);
      mask Display: image(imread('nsi.bmp'));text(0.5, 0.2, 'DigitalOutput_1', 'horizontalAlignment', 'center', 'verticalAlignment', 'base');plot([0.05 0.05 0.05 0.05 0.05 0.05 0.05 0.05 0.05 0.05]);port_label('input', 1, 'H2 : Low Side');
  Init : Subsystem  mask(System Initialize){}
      mask help: Add code to a systems Initialize function
      settings: CopyFcn=cccopyfcn(gcb)  OpenFcn=ccopenfcn('System Initialize Function')
      mask Help: This block contains text fields to insert custom user code sections at the declaration, execution and exit sections of the systems initialize function.  By placing this block inside a subsytem, the custom user code will appear in that subsystems function.
      mask Display: disp('I()')
  Pwm : S-Function  FunctionName=NsiIo_Pwm  Parameters=channel  SFunctionDeploymentMode=off  EnableBusSupport=off  mask(MUXlink I/O Pwm){channel=3}
      mask prompts: channel "Channel ?"
      mask help: Write value onto I/O PWM channel.
      mask init:
      | NsiIo_Pwm_InitializationFcn();
      settings: OpenFcn=NsiIo_Pwm_OpenFcn();
      mask Help:
      | eval('block=get_param(gcb, ''RTWdata'');')
      | web([docroot '\toolbox\MUXlink\html\blocks/' block.MUXlink_BlockType '.html'])
      mask Callback channel: NsiIo_Pwm_ApplyFcn(1);
      mask Display: image(imread('nsi.bmp'));text(0.5, 0.2, 'Pwm_3', 'horizontalAlignment', 'center', 'verticalAlignment', 'base');plot([0.05 0.05 0.05 0.05 0.05 0.05 0.05 0.05 0.05 0.05]);port_label('input', 1, 'Hz');port_label('input', 2, '%');text(0.1, 0.5, 'A1', 'horizontalAlignment','center');
  Pwm1 : S-Function  FunctionName=NsiIo_Pwm  Parameters=channel  SFunctionDeploymentMode=off  EnableBusSupport=off  mask(MUXlink I/O Pwm){channel=2}
      mask prompts: channel "Channel ?"
      mask help: Write value onto I/O PWM channel.
      mask init:
      | NsiIo_Pwm_InitializationFcn();
      settings: OpenFcn=NsiIo_Pwm_OpenFcn();
      mask Help:
      | eval('block=get_param(gcb, ''RTWdata'');')
      | web([docroot '\toolbox\MUXlink\html\blocks/' block.MUXlink_BlockType '.html'])
      mask Callback channel: NsiIo_Pwm_ApplyFcn(1);
      mask Display: image(imread('nsi.bmp'));text(0.5, 0.2, 'Pwm_2', 'horizontalAlignment', 'center', 'verticalAlignment', 'base');plot([0.05 0.05 0.05 0.05 0.05 0.05 0.05 0.05 0.05 0.05]);port_label('input', 1, 'Hz');port_label('input', 2, '%');text(0.1, 0.5, 'E2', 'horizontalAlignment','center');
  Task : S-Function  FunctionName=NsiSys_TaskREF  Parameters=task_initialised,task_periodic, task_sampletime,task_name,task_event,task_offset  SFunctionDeploymentMode=off  EnableBusSupport=off  mask(task definition){task_initialised=on, task_periodic=on, task_sampletime=[0.1], task_offset=0.03, task_name=Hardwired_Outputs, task_event=on}
      mask prompts: task_initialised "task initialised"; task_periodic "Is Periodic"; task_sampletime "Task sample time"; task_offset "Task Offset"; task_name "Task name"; task_event "Is event"
      mask help:
      | Permit to provide all parameters associated to a MUXLINK task.
      | Task can be executed periodicaly and/or on event detection.
      | If task is periodic:
      | Task sample time specify the execution period in mS [0.001   6000]
      | Task Offset specify the offset applied to the execution period
      | Task Offset < Task sample time
      mask init:
      | NsiSys_TaskREF_InitializationFcn();
      settings: OpenFcn=NsiSys_Task_OpenFcn();
      mask Callback task_initialised: NsiSys_TaskREF_ApplyFcn(1);
      mask Callback task_periodic: NsiSys_TaskREF_ApplyFcn(2);
      mask Callback task_sampletime: NsiSys_TaskREF_ApplyFcn(3);
      mask Callback task_offset: NsiSys_TaskREF_ApplyFcn(6);
      mask Callback task_name: NsiSys_TaskREF_ApplyFcn(4);
      mask Callback task_event: NsiSys_TaskREF_ApplyFcn(5);
      mask Display: text(0.5, 0.8, 't()', 'horizontalAlignment', 'center', 'verticalAlignment', 'base');text(0.5, 0.2, '/ 100.0ms / 30.0ms /', 'horizontalAlignment', 'center', 'verticalAlignment', 'base');text(0.5, 0.4, 'Event', 'horizontalAlignment', 'center', 'verticalAlignment', 'base');
  UsbTx : S-Function  FunctionName=NsiUsb_Tx  Parameters=signame,resolution,offset,unite  SFunctionDeploymentMode=off  EnableBusSupport=off  mask(MUXlink Usb Tx){signame=PreCharge, resolution=1, offset=0, unite=}
      mask prompts: signame "Signal name ?"; resolution "Resolution ?"; offset "Offset ?"; unite "Unit ?"
      mask help: Transmit a frame on the USB Channel.
      mask init:
      | NsiUsb_Tx_InitializationFcn();
      settings: OpenFcn=NsiUsb_Tx_OpenFcn();
      mask Help:
      | eval('block=get_param(gcb, ''RTWdata'');')
      | web([docroot '\toolbox\MUXlink\html\blocks/' block.MUXlink_BlockType '.html'])
      mask Callback signame: NsiUsb_Tx_ApplyFcn(1);
      mask Callback resolution: NsiUsb_Tx_ApplyFcn(2);
      mask Callback offset: NsiUsb_Tx_ApplyFcn(3);
      mask Callback unite: NsiUsb_Tx_ApplyFcn(4);
      mask Display: image(imread('nsi.bmp'));text(0.5, 0.2, 'USB Tx', 'horizontalAlignment', 'center', 'verticalAlignment', 'base');plot([0.05 0.05 0.05 0.05 0.05 0.05 0.05 0.05 0.05 0.05]);port_label('input',1, 'PreCharge');
  UsbTx2 : S-Function  FunctionName=NsiUsb_Tx  Parameters=signame,resolution,offset,unite  SFunctionDeploymentMode=off  EnableBusSupport=off  mask(MUXlink Usb Tx){signame=ECU UK, resolution=1, offset=0, unite=Bool}
      mask prompts: signame "Signal name ?"; resolution "Resolution ?"; offset "Offset ?"; unite "Unit ?"
      mask help: Transmit a frame on the USB Channel.
      mask init:
      | NsiUsb_Tx_InitializationFcn();
      settings: OpenFcn=NsiUsb_Tx_OpenFcn();
      mask Help:
      | eval('block=get_param(gcb, ''RTWdata'');')
      | web([docroot '\toolbox\MUXlink\html\blocks/' block.MUXlink_BlockType '.html'])
      mask Callback signame: NsiUsb_Tx_ApplyFcn(1);
      mask Callback resolution: NsiUsb_Tx_ApplyFcn(2);
      mask Callback offset: NsiUsb_Tx_ApplyFcn(3);
      mask Callback unite: NsiUsb_Tx_ApplyFcn(4);
      mask Display: image(imread('nsi.bmp'));text(0.5, 0.2, 'USB Tx', 'horizontalAlignment', 'center', 'verticalAlignment', 'base');plot([0.05 0.05 0.05 0.05 0.05 0.05 0.05 0.05 0.05 0.05]);port_label('input',1, 'ECU UK');
  wires:
  In1/1 -> Bus Selector/1
  Bus Selector/1 -> AnalogOutput1/1  "<Throttle1_Supply>"
  Bus Selector/2 -> AnalogOutput2/1  "<Throttle2_Supply>"
  Bus Selector/5 -> DigitalOutput/1  "<Buzzer>"
  Bus Selector/7 -> DigitalOutput1/1  "<Coolant_Pump>"
  Bus Selector/10 -> Pwm1/2  "<AMS_Light>"
  Bus Selector/3 -> AnalogOutput7/1  "<Pedal_Light>"
  Bus Selector/11 -> UsbTx2/1, AnalogOutput8/1  "<ECU_Ok>"
  Bus Selector/9 -> AnalogOutput6/1, UsbTx/1  "<Pre_Charge>"
  Bus Selector/4 -> AnalogOutput4/1  "<Brake_Supply>"
  Bus Selector/8 -> DigitalOutput2/1  "<Brake_Bool>"
  Bus Selector/6 -> ?  "<MCU_Ground>"
  Constant/1 -> Pwm/1
  Bus Selector/12 -> Pwm/2  "<BSPD_Light>"
  Constant1/1 -> Pwm1/1

== system TBRe18_ECU_V6/High_Priority_CAN_RX ==
  Bus Creator : BusCreator  Inputs=8
  CanRx : S-Function  FunctionName=NsiCan_Rx  Parameters=data_can,channel,msg_name,ident,ident_type,dlc,signals,is_trigger  SFunctionDeploymentMode=off  EnableBusSupport=off  mask(MUXlink Can Rx){data_can=1;HIGH_SPEED;500Kbps;120 Ohm;C:\Users\William\Documents\ECU\DBC\TBRe18_DBC_V1.dbc;0;;1;HIGH_SPEED;500Kbps;120 Ohm;C:\Users\William\Documents\ECU\DBC\TBRe18_DBC_V1.dbc;0;;0;HIGH_SPEED;500Kbps;120 Ohm;C:\Users\l\Desktop\FYP\ECU\DBC\TBRe_DBC_V2.dbc;0;;0;HIGH_SPEED;500Kbps;120 Ohm;D:\TOOLS\MUXLINK\R2011b\MUXlink\misc\j1939_adapt.dbc;0;;0;HIGH_SPEED;1000Kbps;No;D:\TOOLS\MUXLINK\R2011b\MUXlink\misc\BASE_CAN_MUXLAB4.dbc;0;, channel=1, msg_name=MCU_TPDO1, ident=0x181, ident_type=STD, dlc=8, signals=MCU_Torque_Actual_Value;1;40;-16, is_trigger=0}
      mask prompts: data_can "data can"; msg_name "msg name"
      mask help: Receive a frame from a CAN channel.
      mask init:
      | NsiCan_Rx_InitializationFcn();
      settings: OpenFcn=NsiCan_Rx_OpenFcn();
      mask Help:
      | eval('block=get_param(gcb, ''RTWdata'');')
      | web([docroot '\toolbox\MUXlink\html\blocks/' block.MUXlink_BlockType '.html'])
      mask Callback data_can: NsiCan_Rx_ApplyFcn(1);
      mask Callback channel: NsiCan_Rx_ApplyFcn(2);
      mask Callback msg_name: NsiCan_Rx_ApplyFcn(3);
      mask Callback ident: NsiCan_Rx_ApplyFcn(4);
      mask Callback ident_type: NsiCan_Rx_ApplyFcn(5);
      mask Callback dlc: NsiCan_Rx_ApplyFcn(6);
      mask Callback signals: NsiCan_Rx_ApplyFcn(7);
      mask Callback is_trigger: NsiCan_Rx_ApplyFcn(8);
      mask Display: image(imread('nsi.bmp'));text(0.5, 0.3, 'RX_MCU_TPDO1_CAN1', 'horizontalAlignment', 'center', 'verticalAlignment', 'base');plot([0.05 0.05 0.05 0.05 0.05 0.05 0.05 0.05 0.05 0.05]); port_label('output',1, 'MCU_Torque_Actual_Value'); port_label('output',2, 'Status');
  CanRx1 : S-Function  FunctionName=NsiCan_Rx  Parameters=data_can,channel,msg_name,ident,ident_type,dlc,signals,is_trigger  SFunctionDeploymentMode=off  EnableBusSupport=off  mask(MUXlink Can Rx){data_can=1;HIGH_SPEED;500Kbps;120 Ohm;C:\Users\William\Documents\ECU\DBC\TBRe18_DBC_V1.dbc;0;;1;HIGH_SPEED;500Kbps;120 Ohm;C:\Users\William\Documents\ECU\DBC\TBRe18_DBC_V1.dbc;0;;0;HIGH_SPEED;500Kbps;120 Ohm;C:\Users\l\Desktop\FYP\ECU\DBC\TBRe_DBC_V2.dbc;0;;0;HIGH_SPEED;500Kbps;120 Ohm;D:\TOOLS\MUXLINK\R2011b\MUXlink\misc\j1939_adapt.dbc;0;;0;HIGH_SPEED;1000Kbps;No;D:\TOOLS\MUXLINK\R2011b\MUXlink\misc\BASE_CAN_MUXLAB4.dbc;0;, channel=1, msg_name=MCU_TPDO2, ident=0x281, ident_type=STD, dlc=8, signals=Motor_Temp;1;8;8;MCU_Temp;1;0;8;MCU_DC_Link_Voltage;1;16;16, is_trigger=0}
      mask prompts: data_can "data can"; msg_name "msg name"
      mask help: Receive a frame from a CAN channel.
      mask init:
      | NsiCan_Rx_InitializationFcn();
      settings: OpenFcn=NsiCan_Rx_OpenFcn();
      mask Help:
      | eval('block=get_param(gcb, ''RTWdata'');')
      | web([docroot '\toolbox\MUXlink\html\blocks/' block.MUXlink_BlockType '.html'])
      mask Callback data_can: NsiCan_Rx_ApplyFcn(1);
      mask Callback channel: NsiCan_Rx_ApplyFcn(2);
      mask Callback msg_name: NsiCan_Rx_ApplyFcn(3);
      mask Callback ident: NsiCan_Rx_ApplyFcn(4);
      mask Callback ident_type: NsiCan_Rx_ApplyFcn(5);
      mask Callback dlc: NsiCan_Rx_ApplyFcn(6);
      mask Callback signals: NsiCan_Rx_ApplyFcn(7);
      mask Callback is_trigger: NsiCan_Rx_ApplyFcn(8);
      mask Display: image(imread('nsi.bmp'));text(0.5, 0.3, 'RX_MCU_TPDO2_CAN1', 'horizontalAlignment', 'center', 'verticalAlignment', 'base');plot([0.05 0.05 0.05 0.05 0.05 0.05 0.05 0.05 0.05 0.05]); port_label('output',1, 'Motor_Temp'); port_label('output',2, 'MCU_Temp'); port_label('output',3, 'MCU_DC_Link_Voltage'); port_label('output',4, 'Status');
  CanRx2 : S-Function  FunctionName=NsiCan_Rx  Parameters=data_can,channel,msg_name,ident,ident_type,dlc,signals,is_trigger  SFunctionDeploymentMode=off  EnableBusSupport=off  mask(MUXlink Can Rx){data_can=1;HIGH_SPEED;500Kbps;120 Ohm;C:\Users\William\Documents\ECU\DBC\TBRe18_DBC_V1.dbc;0;;1;HIGH_SPEED;500Kbps;120 Ohm;C:\Users\William\Documents\ECU\DBC\TBRe18_DBC_V1.dbc;0;;0;HIGH_SPEED;500Kbps;120 Ohm;C:\Users\l\Desktop\FYP\ECU\DBC\TBRe_DBC_V2.dbc;0;;0;HIGH_SPEED;500Kbps;120 Ohm;D:\TOOLS\MUXLINK\R2011b\MUXlink\misc\j1939_adapt.dbc;0;;0;HIGH_SPEED;1000Kbps;No;D:\TOOLS\MUXLINK\R2011b\MUXlink\misc\BASE_CAN_MUXLAB4.dbc;0;, channel=1, msg_name=MCU_SDO_Response, ident=0x581, ident_type=STD, dlc=8, signals=SDO_Response_Command;1;0;8;MCU_OD_Sub_Index;1;24;8;MCU_OD_Index;1;8;16;SDO_Data;1;32;32, is_trigger=0}
      mask prompts: data_can "data can"; msg_name "msg name"
      mask help: Receive a frame from a CAN channel.
      mask init:
      | NsiCan_Rx_InitializationFcn();
      settings: OpenFcn=NsiCan_Rx_OpenFcn();
      mask Help:
      | eval('block=get_param(gcb, ''RTWdata'');')
      | web([docroot '\toolbox\MUXlink\html\blocks/' block.MUXlink_BlockType '.html'])
      mask Callback data_can: NsiCan_Rx_ApplyFcn(1);
      mask Callback channel: NsiCan_Rx_ApplyFcn(2);
      mask Callback msg_name: NsiCan_Rx_ApplyFcn(3);
      mask Callback ident: NsiCan_Rx_ApplyFcn(4);
      mask Callback ident_type: NsiCan_Rx_ApplyFcn(5);
      mask Callback dlc: NsiCan_Rx_ApplyFcn(6);
      mask Callback signals: NsiCan_Rx_ApplyFcn(7);
      mask Callback is_trigger: NsiCan_Rx_ApplyFcn(8);
      mask Display: image(imread('nsi.bmp'));text(0.5, 0.3, 'RX_MCU_SDO_Response_CAN1', 'horizontalAlignment', 'center', 'verticalAlignment', 'base');plot([0.05 0.05 0.05 0.05 0.05 0.05 0.05 0.05 0.05 0.05]); port_label('output',1, 'SDO_Response_Command'); port_label('output',2, 'MCU_OD_Sub_Index'); port_label('output',3, 'MCU_OD_Index'); port_label('output',4, 'SDO_Data'); port_label('output',5, 'Status');
  Init : Subsystem  mask(System Initialize){}
      mask help: Add code to a systems Initialize function
      settings: CopyFcn=cccopyfcn(gcb)  OpenFcn=ccopenfcn('System Initialize Function')
      mask Help: This block contains text fields to insert custom user code sections at the declaration, execution and exit sections of the systems initialize function.  By placing this block inside a subsytem, the custom user code will appear in that subsystems function.
      mask Display: disp('I()')
  Task : S-Function  FunctionName=NsiSys_TaskREF  Parameters=task_initialised,task_periodic, task_sampletime,task_name,task_event,task_offset  SFunctionDeploymentMode=off  EnableBusSupport=off  mask(task definition){task_initialised=on, task_periodic=on, task_sampletime=[0.1], task_offset=0.03, task_name=High_Priority_CAN_RX, task_event=on}
      mask prompts: task_initialised "task initialised"; task_periodic "Is Periodic"; task_sampletime "Task sample time"; task_offset "Task Offset"; task_name "Task name"; task_event "Is event"
      mask help:
      | Permit to provide all parameters associated to a MUXLINK task.
      | Task can be executed periodicaly and/or on event detection.
      | If task is periodic:
      | Task sample time specify the execution period in mS [0.001   6000]
      | Task Offset specify the offset applied to the execution period
      | Task Offset < Task sample time
      mask init:
      | NsiSys_TaskREF_InitializationFcn();
      settings: OpenFcn=NsiSys_Task_OpenFcn();
      mask Callback task_initialised: NsiSys_TaskREF_ApplyFcn(1);
      mask Callback task_periodic: NsiSys_TaskREF_ApplyFcn(2);
      mask Callback task_sampletime: NsiSys_TaskREF_ApplyFcn(3);
      mask Callback task_offset: NsiSys_TaskREF_ApplyFcn(6);
      mask Callback task_name: NsiSys_TaskREF_ApplyFcn(4);
      mask Callback task_event: NsiSys_TaskREF_ApplyFcn(5);
      mask Display: text(0.5, 0.8, 't()', 'horizontalAlignment', 'center', 'verticalAlignment', 'base');text(0.5, 0.2, '/ 100.0ms / 30.0ms /', 'horizontalAlignment', 'center', 'verticalAlignment', 'base');text(0.5, 0.4, 'Event', 'horizontalAlignment', 'center', 'verticalAlignment', 'base');
  Out1 : Outport
  wires:
  Bus Creator/1 -> Out1/1
  CanRx/1 -> Bus Creator/1  "MCU_Target_Torque"
  CanRx2/1 -> Bus Creator/2  "SDO_Response_Command"
  CanRx2/2 -> Bus Creator/3  "OD_Sub_Index"
  CanRx2/3 -> Bus Creator/4  "OD_Index"
  CanRx2/4 -> Bus Creator/5  "SDO_Data"
  CanRx1/1 -> Bus Creator/6  "Motor_Temp"
  CanRx1/2 -> Bus Creator/7  "MCU_Temp"
  CanRx1/3 -> Bus Creator/8  "MCU_DC_Link_Voltage"
